simulink model "Boost_convert2"  (R2017a)
settings: Solver=ode45  StartTime=0.0  StopTime=10.0  RelTol=1e-3  EnableMultiTasking=on
libraries: powerlib x12
settings Model: Creator=radow  LastModifiedBy=radow
settings DataIOCC: LimitDataPoints=on  SaveFormat=Array
settings OptimizationCC: LifeSpan=inf
settings DebuggingCC: UnderspecifiedInitializationDetection=Classic  MergeDetectMultiDrivingBlocksExec=none  SolverPrmCheckMsg=warning  StateNameClashWarn=warning  SFUnexpectedBacktrackingDiag=warning  SFNoUnconditionalDefaultTransitionDiag=warning  SFExecutionAtInitializationDiag=none
settings HardwareCC: ProdBitPerPointer=32  ProdBitPerSizeT=32  ProdBitPerPtrDiffT=32  ProdLargestAtomicFloat=None  ProdIntDivRoundTo=Undefined  ProdEndianess=Unspecified  ProdWordSize=32  ProdHWDeviceType=32-bit Generic
settings ModelReferenceCC: PropagateSignalLabelsOutOfModel=off
settings GRTTargetCC: TargetLangStandard=C89/C90 (ANSI)  GeneratePreprocessorConditionals=Disable all
settings ConfigComp: CovMetricSettings=dw  CovHtmlReporting=on  CovSaveCumulativeToWorkspaceVar=on  CovSaveSingleToWorkspaceVar=on  CovExternalEMLEnable=off

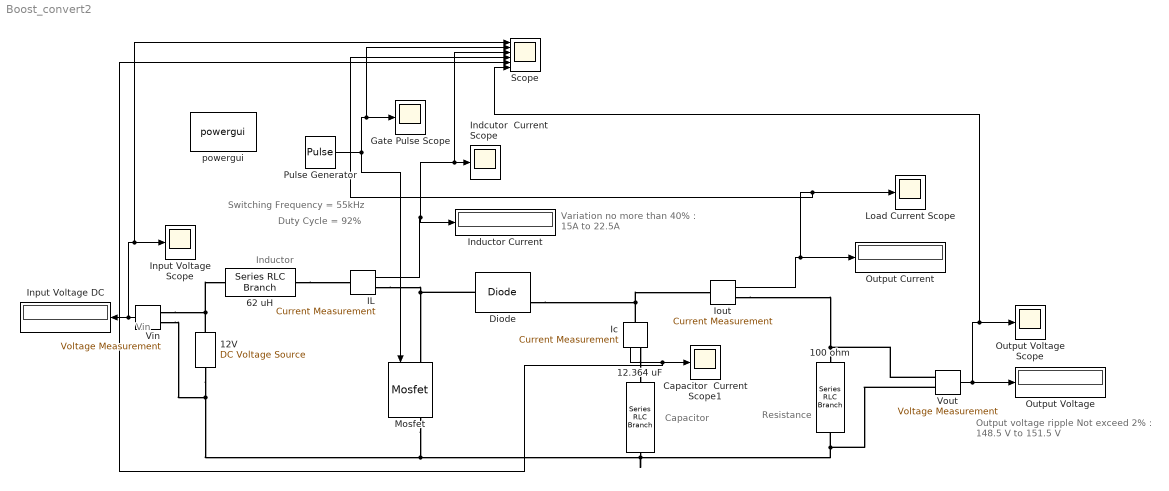
== system Boost_convert2 ==
  note: Vin
  note: Output voltage ripple Not exceed 2% :
      | 148.5 V to 151.5 V
  note: Variation no more than 40% :
      | 15A to 22.5A
  note: Duty Cycle = 92%
  note: Switching Frequency = 55kHz
  note: Resistance
  note: Capacitor
  note: Inductor
  100 ohm : powerlib/Elements/Series RLC Branch  LConnTagsString=__new0  RConnTagsString=__new0  BranchType=R  Resistance=100  Inductance=1e-3  SetiL0=off  InitialCurrent=0  Capacitance=1e-6  Setx0=off  InitialVoltage=0  Measurements=None
  12.364 uF : powerlib/Elements/Series RLC Branch  LConnTagsString=__new0  RConnTagsString=__new0  BranchType=C  Resistance=1  Inductance=1e-3  SetiL0=off  InitialCurrent=0  Capacitance=500.84e-6  Setx0=off  InitialVoltage=0  Measurements=None
  12V : powerlib/Electrical Sources/DC Voltage Source  Amplitude=12  Measurements=None
  62 uH : powerlib/Elements/Series RLC Branch  LConnTagsString=__new0  RConnTagsString=__new0  BranchType=L  Resistance=1  Inductance=0.544e-3  SetiL0=off  InitialCurrent=0  Capacitance=1e-6  Setx0=off  InitialVoltage=0  Measurements=None
  Capacitor  Current Scope1 : Scope
  Diode : powerlib/Power Electronics/Diode  Ron=0.00001  Lon=0  Vf=0  IC=0  UseSnubber=off  Rs=0  Cs=0  Measurements=on
  Gate Pulse Scope : Scope
  IL : powerlib/Measurements/Current Measurement  PhasorSimulation=off  OutputType=Complex  PSBequivalent=0
  Ic : powerlib/Measurements/Current Measurement  PhasorSimulation=off  OutputType=Complex  PSBequivalent=0
  Indcutor  Current Scope : Scope
  Inductor Current : Display
  Input Voltage DC : Display
  Input Voltage Scope : Scope
  Iout : powerlib/Measurements/Current Measurement  PhasorSimulation=off  OutputType=Complex  PSBequivalent=0
  Load Current Scope : Scope
  Mosfet : powerlib/Power Electronics/Mosfet  Ron=0.0001  Lon=0  Rd=0.001  Vfd=0  IC=0  Rs=500  Cs=inf  Measurements=on
  Output Current : Display
  Output Voltage : Display
  Output Voltage Scope : Scope
  Pulse Generator : DiscretePulseGenerator  PulseType=Time based  Period=1/6000  PulseWidth=92
  Scope : Scope  NumInputPorts=6
  Vin : powerlib/Measurements/Voltage Measurement  PhasorSimulation=off  OutputType=Complex  PSBequivalent=0
  Vout : powerlib/Measurements/Voltage Measurement  PhasorSimulation=off  OutputType=Complex  PSBequivalent=0
  powergui : powerlib/powergui  Priority=1  SimulationMode=Continuous  SampleTime=50e-6  frequency=60  Iterations=50  frequencyindice=0  Pbase=100e6  ErrMax=1e-4  UnitsV=kV  UnitsW=MW  buscounter=0  FunctionMessages=off  echomessages=off  EnableUseOfTLC=off  CurrentSourceSwitches=off  DisableSnubberDevices=off  DisableRonSwitches=off  DisableVfSwitches=off  DisplayEquations=off  SolverType=Tustin  Interpol=off  ExternalGateDelay=off  methode=off  Ts=0  x0status=blocks  SPID=off  SwTol=0  HookPort=off  RestoreLinks=warning  ResistiveCurrentMeasurement=off  Frange=[0:2:500]  Ylog=off  Xlog=on  ShowGrid=off  save=off  variable=ZData  structure=0  ZoomFFT=off  StartTime=0.0  cycles=1  DisplayStyle=1  fundamental=60  FreqAxis=off  MaxFrequency=1000  frequencyindicesteady=1  RmsSteady=1  display=off
  wires:
  Vout/1 -> Scope/6, Output Voltage Scope/1, Output Voltage/1
  Pulse Generator/1 -> Mosfet/1, Scope/2, Gate Pulse Scope/1
  Vin/1 -> Scope/1, Input Voltage Scope/1, Input Voltage DC/1
  Iout/1 -> Scope/4, Load Current Scope/1, Output Current/1
  IL/1 -> Scope/3, Indcutor  Current Scope/1, Inductor Current/1
  Ic/1 -> Scope/5, Capacitor  Current Scope1/1
  connections:
  Ic/LConn1 -- Diode/RConn1 -- Iout/LConn1
  100 ohm/RConn1 -- Vout/LConn2 -- 12.364 uF/RConn1 -- Vin/LConn2 -- 12V/LConn1 -- Mosfet/RConn1
  Iout/RConn1 -- Vout/LConn1 -- 100 ohm/LConn1
  12V/RConn1 -- Vin/LConn1 -- 62 uH/LConn1
  IL/RConn1 -- Diode/LConn1 -- Mosfet/LConn1
  Ic/RConn1 -- 12.364 uF/LConn1
  62 uH/RConn1 -- IL/LConn1
